simulink model "fixedWingPathFollowing"  (R2021a)
settings: Solver=VariableStepAuto  StartTime=0.0  StopTime=1600  FixedStep=0.01  RelTol=1e-3
libraries: robotcorelib x1, uavutilslib x1
settings Model: DataDictionary=fixedWingPathFollowingData.sldd  EnableAccessToBaseWorkspace=off  EnablePacing=on  PacingRate=10  Creator=The MathWorks, Inc.  LastModifiedBy=hgu8
settings SolverCC: AlgebraicLoopSolver=TrustRegion  DecoupledContinuousIntegration=on
settings DataIOCC: ReturnWorkspaceOutputs=off
settings OptimizationCC: UseDivisionForNetSlopeComputation=UseDivisionForReciprocalsOfIntegersOnly
settings DebuggingCC: SFMachineParentedDataDiag=warning  ArithmeticOperatorsInVariantConditions=warning
settings SFSimCC: SimUseLocalCustomCode=off  CustomCodeUndefinedFunction=UseInterfaceOnly
settings RTWCC: RTWUseLocalCustomCode=off

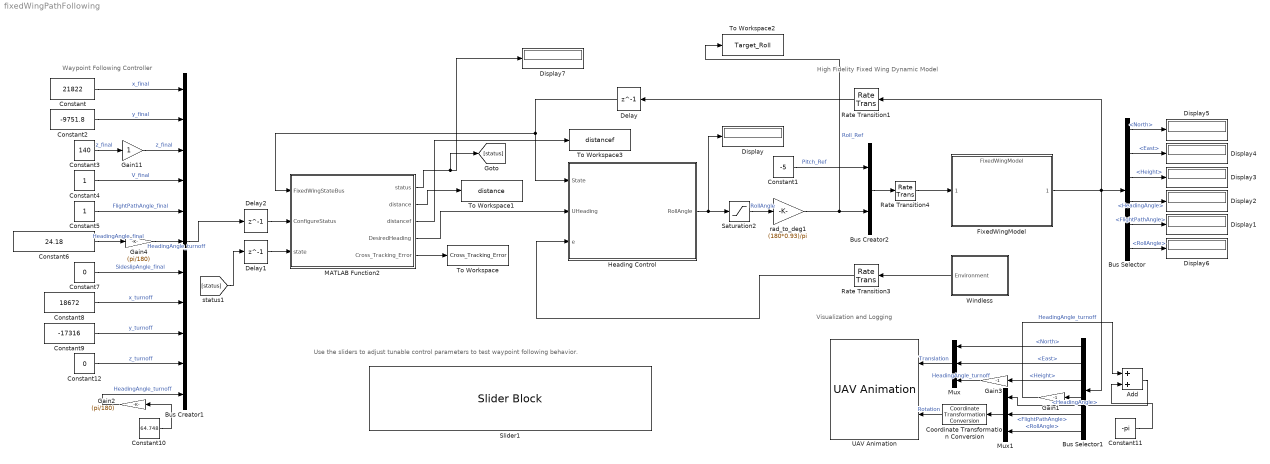
== system fixedWingPathFollowing ==
  note: Use the sliders to adjust tunable control parameters to test waypoint following behavior.
  note: Visualization and Logging
  note: High Fidelity Fixed Wing Dynamic Model
  note: Waypoint Following Controller
  Add : Sum
  Bus Creator1 : BusCreator  Inputs=11  OutDataTypeStr=Bus: ConfigureStatus
  Bus Creator2 : BusCreator  Inputs=2  OutDataTypeStr=Bus: FixedWingControlBus2  NonVirtualBus=on
  Bus Selector : BusSelector  OutputSignals=North,East,Height,HeadingAngle,FlightPathAngle,RollAngle
  Bus Selector1 : BusSelector  OutputSignals=North,East,Height,HeadingAngle,FlightPathAngle,RollAngle
  Constant : Constant  Value=21822
  Constant1 : Constant  Value=-5
  Constant10 : Constant  Value=64.748
  Constant11 : Constant  Value=-pi
  Constant12 : Constant  Value=0
  Constant2 : Constant  Value=-9751.8  VectorParams1D=off
  Constant3 : Constant  Value=140
  Constant4 : Constant
  Constant5 : Constant
  Constant6 : Constant  Value=24.18
  Constant7 : Constant  Value=0
  Constant8 : Constant  Value=18672
  Constant9 : Constant  Value=-17316
  Coordinate Transformation Conversion : robotcorelib/Coordinate Transformation Conversion  InputRepresentation=Euler Angles  InputEulerSequence=ZYX  ShowTrVecInputPort=on  OutputRepresentation=Quaternion  OutputEulerSequence=ZYX  ShowTrVecOutputPort=on  SimulateUsing=Code generation
      settings: SourceProductBaseCode=NV,RO,RR,UV
  Delay : Delay  DelayLength=1  InitialCondition=0
  Delay1 : Delay  DelayLength=1  InitialCondition=0
  Delay2 : Delay  DelayLength=1  InitialCondition=0
  Display{,1..7} (8 alike) : Display
  FixedWingModel : ModelReference  ModelNameDialog=FixedWingModel.slx  SimulationMode=Normal  ModelReferenceVersion=3.53
  Gain1 : Gain  Gain=-1
  Gain11 : Gain
  Gain2 : Gain  Gain=(pi/180)
  Gain3 : Gain  Gain=-1
  Gain4 : Gain  Gain=(pi/180)
  Heading Control : MATLAB Function  TreatAsAtomicUnit=on  mask(Fixed Wing Heading Controller){PHeadingAngle=0.39}
      mask prompts: PHeadingAngle "Heading Control Gain"
      mask help: P controller that regulates fixed wing UAV heading direction through controlling its roll angle. This controller requires that the plane is flying under coordinated flight condition.
  MATLAB Function2 : MATLAB Function  TreatAsAtomicUnit=on
  Mux : Mux  Inputs=3
  Mux1 : Mux  Inputs=3
  Rate Transition1 : RateTransition  OutPortSampleTime=0.01
  Rate Transition3 : RateTransition  OutPortSampleTime=0.01
  Rate Transition4 : RateTransition  OutPortSampleTime=0.1
  Saturation2 : Saturate  UpperLimit=20*pi/180  LowerLimit=-20*pi/180
  Slider1 : SliderBlock  ScaleMin=0.39000000000000001  ScaleMax=3.8999999999999999
  To Workspace : ToWorkspace  VariableName=Cross_Tracking_Error  SaveFormat=Timeseries  SampleTime=-1
  To Workspace1 : ToWorkspace  VariableName=distance  SaveFormat=Timeseries  SampleTime=-1
  To Workspace2 : ToWorkspace  VariableName=Target_Roll  SaveFormat=Timeseries  SampleTime=-1
  To Workspace3 : ToWorkspace  VariableName=distancef  SaveFormat=Timeseries  SampleTime=-1
  UAV Animation : uavutilslib/UAV Animation  UAVType=FixedWing  UAVSize=50  InertialZDirection=Down  SampleTime=0.01
      settings: SourceProductBaseCode=UV
  Windless : Subsystem  VariantControl=NoWind
  rad_to_deg1 : Gain  Gain=(180*0.93)/pi
  wires:
  Saturation2/1 -> rad_to_deg1/1  "RollAngle"
  Bus Selector1/3 -> Gain3/1  "<Height>"
  Bus Selector1/6 -> Mux1/3  "<RollAngle>"
  Mux1/1 -> Coordinate Transformation Conversion/1
  Coordinate Transformation Conversion/1 -> UAV Animation/2  "Rotation"
  Mux/1 -> UAV Animation/1  "Translation"
  Windless/1(Environment) -> Rate Transition3/1
  Rate Transition3/1 -> Heading Control/3(e)
  Bus Creator2/1 -> Rate Transition4/1
  rad_to_deg1/1 -> To Workspace2/1, Bus Creator2/2  "Roll_Ref"
  Constant1/1 -> Bus Creator2/1  "Pitch_Ref"
  Rate Transition1/1 -> Delay/1
  Rate Transition4/1 -> FixedWingModel/1
  FixedWingModel/1 -> Bus Selector1/1, Bus Selector/1, Rate Transition1/1
  Constant12/1 -> Bus Creator1/10  "z_turnoff"
  [status] -> Delay1/1
  Constant4/1 -> Bus Creator1/4  "V_final"
  Constant7/1 -> Bus Creator1/7  "SideslipAngle_final"
  MATLAB Function2/1(status) -> Display7/1, [status]
  Constant5/1 -> Bus Creator1/5  "FlightPathAngle_final"
  Bus Creator1/1 -> Delay2/1
  Constant/1 -> Bus Creator1/1  "x_final"
  Constant3/1 -> Gain11/1  "z_final"
  Constant2/1 -> Bus Creator1/2  "y_final"
  MATLAB Function2/4(DesiredHeading) -> Heading Control/2(UHeading)
  Constant8/1 -> Bus Creator1/8  "x_turnoff"
  Constant6/1 -> Gain4/1  "HeadingAngle_final"
  Gain11/1 -> Bus Creator1/3  "z_final"
  MATLAB Function2/2(distance) -> To Workspace1/1
  Constant10/1 -> Gain2/1
  Delay/1 -> MATLAB Function2/1(FixedWingStateBus), Heading Control/1(State)
  Delay1/1 -> MATLAB Function2/3(state)
  Delay2/1 -> MATLAB Function2/2(ConfigureStatus)
  MATLAB Function2/5(Cross_Tracking_Error) -> To Workspace/1
  Bus Selector/1 -> Display5/1  "<North>"
  Bus Selector/2 -> Display4/1  "<East>"
  Bus Selector/3 -> Display3/1  "<Height>"
  Bus Selector/4 -> Display2/1  "<HeadingAngle>"
  Bus Selector/5 -> Display1/1  "<FlightPathAngle>"
  Bus Selector/6 -> Display6/1  "<RollAngle>"
  Constant9/1 -> Bus Creator1/9  "y_turnoff"
  Heading Control/1(RollAngle) -> Saturation2/1, Display/1
  Bus Selector1/5 -> Mux1/2  "<FlightPathAngle>"
  Gain2/1 -> Bus Creator1/11  "HeadingAngle_turnoff"
  Bus Selector1/4 -> Gain1/1  "<HeadingAngle>"
  Bus Selector1/1 -> Mux/1  "<North>"
  Bus Selector1/2 -> Mux/2  "<East>"
  MATLAB Function2/3(distancef) -> To Workspace3/1
  Gain1/1 -> Add/1  "HeadingAngle_turnoff"
  Constant11/1 -> Add/2
  Add/1 -> Mux1/1
  Gain3/1 -> Mux/3  "HeadingAngle_turnoff"
  Gain4/1 -> Bus Creator1/6  "HeadingAngle_turnoff"

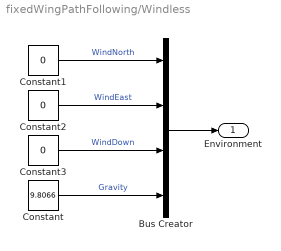
== system fixedWingPathFollowing/Windless ==
  Bus Creator : BusCreator  Inputs=4  OutDataTypeStr=Bus: FixedWingEnvironmentBus  NonVirtualBus=on
  Constant : Constant  Value=9.8066
  Constant1 : Constant  Value=0
  Constant2 : Constant  Value=0
  Constant3 : Constant  Value=0
  Environment : Outport  VectorParamsAs1DForOutWhenUnconnected=off
  wires:
  Constant2/1 -> Bus Creator/2  "WindEast"
  Constant3/1 -> Bus Creator/3  "WindDown"
  Constant1/1 -> Bus Creator/1  "WindNorth"
  Bus Creator/1 -> Environment/1
  Constant/1 -> Bus Creator/4  "Gravity"

== matlab function fixedWingPathFollowing/MATLAB Function2 ==
  data: status output; distance output; distancef output; DesiredHeading output; FixedWingStateBus input; ConfigureStatus input; state input; Cross_Tracking_Error output
function [status, distance, distancef, DesiredHeading,Cross_Tracking_Error] = Waypoint_Follower(FixedWingStateBus,ConfigureStatus,state)

%% before running this planning algorithm, You are suppose to test trjectory following algorithm at three different status invidsually so that adjust parameters in while condition.

    % initialize some variable to avoid the bug not fully defined on execuation
    % path   
    DesiredHeading = 0;
    Cross_Tracking_Error = 0;
    % Current and Final states %
    xi     =   FixedWingStateBus.North;          % Current x-axis position (m)
    yi     =   FixedWingStateBus.East;          % Current y-axis position (m)
    zi     =   FixedWingStateBus.Height;          % Current z-axis position (m)
    %Vi     =   FlightState.V;          % Current forward velocity (m/s)
    gammai =   FixedWingStateBus.FlightPathAngle;          % Current flight path angle (rad)
    psii   =   atan2(sin(FixedWingStateBus.HeadingAngle) , cos(FixedWingStateBus.HeadingAngle));          % Current heading angle phi (rad)
    betai  =   0;          % Current sideslip angle (rad)

    xf     =   ConfigureStatus.x_final;          % Final x-axis position (ft)
    yf     =   ConfigureStatus.y_final;          % Final y-axis position (ft)
    zf     =   ConfigureStatus.z_final;         % Final z-axis position (ft)
    Vf     =   ConfigureStatus.V_final;         % Final forward velocity (ft/s)
    gammaf =   ConfigureStatus.FlightPathAngle_final;         % Final flight path angle (rad)
    psif   =   atan2(sin(ConfigureStatus.HeadingAngle_final) , cos(ConfigureStatus.HeadingAngle_final));         % Final heading angle phi (rad)
    betaf  =   ConfigureStatus.SideslipAngle_final;         % Final sideslip angle (rad)

    % Positon Where engine is broken
    xb     =   ConfigureStatus.x_turnoff;
    yb     =   ConfigureStatus.y_turnoff;
    zb     =   ConfigureStatus.z_turnoff; 
    psib   =   atan2(sin(ConfigureStatus.HeadingAngle_turnoff) , cos(ConfigureStatus.HeadingAngle_turnoff)); % convert range (0~360) to (-pi~pi)
    % Mission phase
    status =   state;         % Mission phase

    %%
    Rl         =   1016;                                  % Loiter radius (m)
    xl         =   xf + 7 * Rl * cos(psif - pi);          % Shifting the x-axis center of loitering 
    yl         =   yf + 7 * Rl * sin(psif - pi);          % Shifting the x-axis center of loitering
    xu         =   xl + Rl * cos(psif - pi);
    yu         =   yl + Rl * sin(psif - pi);
    
    distance   =   sqrt((xi-xl)^2+(yi-yl)^2);             % Distance to loitering center
    % Call function for conducting planned path
    distancef  =   sqrt((xi-xf)^2+(yi-yf)^2);
    za = 1000;
    
    if(distance > 2000 && zi>za)    %  Cruise mode: Far away from landing site %% if condition has problem
        
        status = 1;

%% Parameters for Straight Line Chasing
delta = 1000; %distance of the look ahead point
W_i = [0 0];%straight line origin
W_ip1 = [(xl-xb) (yl-yb)];  %straight line destination
%^^^^^^^^^^^^^^^^^^^^^Update UAV movements^^^^^^^^^^^^^^^^^^^^^^^^^
P_new = [(xi-xb) (yi-yb) zi];
psi_new = psii;
%% consider to replace P_new with a real time position
%if(P_new(1)>W_ip1(1) && P_new(2)>W_ip1(2))
if(distance>2000 && zi>za)
% while condition is up to broken position and final landing position, before defining it, do test program first.

path_g = abs (((P_new(1) - W_i(1))^2) + ((P_new(2) - W_i(2))^2)) ^(1/2); %Calculation of UAV distance from origin
theta = atan2((W_ip1(2)-W_i(2)),(W_ip1(1)-W_i(1))); %path angle calculation
thetau = atan2((P_new(2)-W_i(2)),P_new(1)-W_i(1));  %UAV path angle from origin

l_d=theta-thetau;
Ru=((path_g^2)-((path_g*sin(l_d))^2))^(1/2);
%^^^^^^^^^^^^^^^^^^^^^^Definition of the look ahead point^^^^^^^^^^^^^^^^^^
x_i = ((Ru)+delta)*(cos(theta));
y_i = ((Ru)+delta)*(sin(theta));
p_i = [x_i y_i];
psi_d = atan2((y_i-(P_new(2))),(x_i-(P_new(1)))); %calculation of desired heading angle
    
if psi_d >=0
   DesiredHeading = -psi_d-pi;
elseif psi_d < 0
   DesiredHeading = -(psi_d + 2*pi)-pi;
end

Cross_Tracking_Error = (abs(Ru^2 - path_g^2))^(1/2);

end
                     


    elseif(distance<2000 && zi>za)      % Loiter mode: Close to the landing site, but a high altitude
       
       status = 2; 

%% Parameters for loiter Chasing %%
    r = 1016; %radius of loiter curve(for test need we customize the radius, the actual value is loiter radius)
    %O = [xb 1500+yb]; %center of loiter or circular orbit(for test need we customize the loiter center, the actual loiter center is loiter center calculated before)
    O = [xl yl];
    delta = 0.3; %look ahead position
%^^^^^^^^^^^^^^^^^^^^^Update UAV movements^^^^^^^^^^^^^^^^^^^^^^^^^
    %P_new = [FixedWingStateBus.North FixedWingStateBus.East FixedWingStateBus.Height];
    P_new = [xi yi 0];
    psi_new = psii;

    if (distance<2000 && zi>za)
    Ru = abs ((((P_new(1) - O(1))^2) + ((P_new(2) - O(2))^2)) ^(1/2)-r);%Calculation of UAV distance from center
    theta_new = atan2((P_new(2)-O(2)),(P_new(1)-O(1))); %new path angle calculation
    x_i = ((r*(cos(theta_new+delta)))+O(1));
    y_i = ((r*(sin(theta_new+delta)))+O(2));
    psi_d = atan2((y_i-P_new(2)),(x_i-P_new(1)));%calculation of desired heading angle
    %Desired Heading Angle is very important!!!it is different with that of
    %low fidelity test program.
    if psi_d >=0
       DesiredHeading = -psi_d-pi;
    elseif psi_d < 0
       DesiredHeading = -(psi_d + 2*pi)-pi;
    end

    Cross_Tracking_Error = (abs(((O(1)-P_new(1))^2)+((O(2)-P_new(2))^2))^(1/2))-r;
    end

%}

   else           % Approach to the landing strip
     
               
%% Parameters for Straight Line Chasing
    delta = 1000; %distance of the look ahead point
    W_i = [0 0]; %straight line origin
    W_ip1 = [(xf-xu) (yf-yu)]; %straight line destination suggestion!!! set y coordinate of reference line as zero to reduce the cross tracking error

%^^^^^^^^^^^^^^^^^^^^^Update UAV movements^^^^^^^^^^^^^^^^^^^^^^^^^
   %P_new = [(xi-xb) (yi-yb) zi];%() is very important!
 
   P_new = [(xi-xu) (yi-yu) zi];
   psi_new = psii;  
   %% consider to replace P_new with a real time position
  % if (P_new(1)<W_ip1(1) && P_new(1)<W_ip1(2))
   if (zi<za)
   status = 3;  

   path_g = abs (((P_new(1) - W_i(1))^2) + ((P_new(2) - W_i(2))^2)) ^(1/2); %Calculation of UAV distance from origin
   theta = atan2((W_ip1(2)-W_i(2)),(W_ip1(1)-W_i(1))); %path angle calculation
   thetau = atan2((P_new(2)-W_i(2)),P_new(1)-W_i(1));%UAV path angle from origin

   l_d=theta-thetau;
   Ru=((path_g^2)-((path_g*sin(l_d))^2))^(1/2);
%^^^^^^^^^^^^^^^^^^^^^^Definition of the look ahead point^^^^^^^^^^^^^^^^^^
   x_i = ((Ru)+delta)*(cos(theta));
   y_i = ((Ru)+delta)*(sin(theta));
   p_i = [x_i y_i];
   psi_d = atan2((y_i-(P_new(2))),(x_i-(P_new(1)))); %calculation of desired heading angle
    
    if psi_d >=0
       DesiredHeading = -psi_d-pi;
    elseif psi_d < 0
       DesiredHeading = -(psi_d + 2*pi)-pi;
    end
   Cross_Tracking_Error = (abs(Ru^2 - path_g^2))^(1/2);
        
    end
   
    end
end

== matlab function fixedWingPathFollowing/Heading Control ==
  data: State input Bus: FixedWingStateBus; UHeading input; RollAngle output size=[1 1]; e input Bus: FixedWingEnvironmentBus; PHeadingAngle parameter
function RollAngle = fcn(State, UHeading, e, PHeadingAngle)
    
    Va = State.AirSpeed;
    HeadingAngle = State.HeadingAngle;
    FlightPathAngle = State.FlightPathAngle;
    
    YawAngle = HeadingAngle - asin((1/Va)*[e.WindNorth, e.WindEast]*[-sin(HeadingAngle); cos(HeadingAngle)]);
    b = [cos(HeadingAngle)*cos(FlightPathAngle), sin(HeadingAngle)*cos(FlightPathAngle), -sin(FlightPathAngle)]*[e.WindNorth; e.WindEast; e.WindDown];
    c = [e.WindNorth, e.WindEast, e.WindDown]*[e.WindNorth; e.WindEast; e.WindDown]- Va^2;
    Vg = -b+sqrt(b^2-c);
    
    RollAngle = atan2(PHeadingAngle*angdiff(HeadingAngle,UHeading)*Vg,e.Gravity*cos(HeadingAngle-YawAngle));
